simulink model "iopid_manually_tunning"  (R2017b)
settings: Solver=FixedStepAuto  StartTime=0.0  StopTime=100  FixedStep=0.01  RelTol=1e-3
undefined symbols (not defined in the file): CoordinateFrame, TypeMask, Velocity
libraries: robotlib x3, simulink x1
settings Model: Creator=bshang2  LastModifiedBy=bshang2
settings CodeAppCC: StateflowObjectComments=on

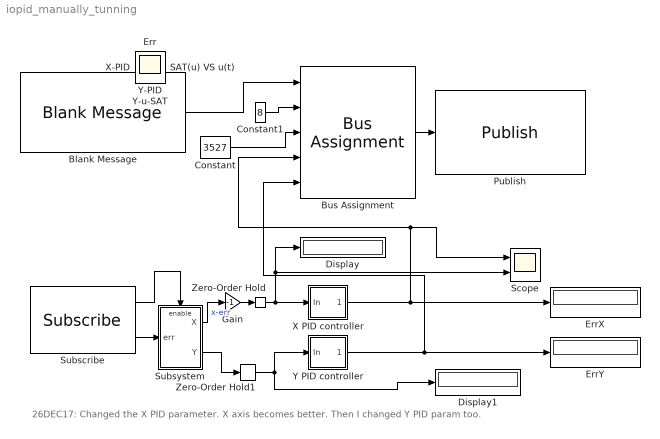
== system iopid_manually_tunning ==
  note: 26DEC17: Changed the X PID parameter. X axis becomes better. Then I changed Y PID param too.
  Blank Message : robotlib/Blank Message  SourceLibraryInfo=This block requires Robotics System Toolbox  messageType=mavros_msgs/PositionTarget  SampleTime=inf
      settings: SourceProductBaseCode=RO
  Bus Assignment : BusAssignment  AssignedSignals=CoordinateFrame,TypeMask,Velocity.X,Velocity.Y
  Constant : Constant  Value=3527  OutDataTypeStr=uint16
  Constant1 : Constant  Value=8  OutDataTypeStr=uint8
  Display : Display
  Display1 : Display
  ErrX : Display
  ErrY : Display
  Gain : Gain  Gain=-1
  Publish : robotlib/Publish  SourceLibraryInfo=This block requires Robotics System Toolbox  topicSource=Select from ROS network  topic=/mavros/setpoint_raw/local  messageType=mavros_msgs/PositionTarget  messageQueueLength=1
      settings: SourceProductBaseCode=RO
  Scope : Scope  NumInputPorts=2
  Subscribe : robotlib/Subscribe  SourceLibraryInfo=This block requires Robotics System Toolbox  topicSource=Select from ROS network  topic=/matlab/err  messageType=geometry_msgs/Pose2D  sampleTime=-1  messageQueueLength=1
      settings: SourceProductBaseCode=RO
  Subsystem : Subsystem
  X PID controller : Subsystem
  Y PID controller : Subsystem
  Zero-Order Hold : ZeroOrderHold  SampleTime=-1
  Zero-Order Hold1 : ZeroOrderHold  SampleTime=-1
  Err : Scope
  SAT(u) VS u(t) : Scope
  X-PID : Scope
  Y-PID : Scope
  Y-u-SAT : Scope
  wires:
  Blank Message/1 -> Bus Assignment/1
  X PID controller/1(Out) -> ErrX/1, Scope/1, Bus Assignment/4
  Bus Assignment/1 -> Publish/1
  Subscribe/2 -> Subsystem/1(err)
  Subsystem/1(X) -> Gain/1  "x-err"
  Subsystem/2(Y) -> Zero-Order Hold1/1
  Subscribe/1 -> Subsystem/Enable
  Y PID controller/1(Out) -> Bus Assignment/5, ErrY/1
  Constant/1 -> Bus Assignment/3
  Constant1/1 -> Bus Assignment/2
  Zero-Order Hold/1 -> Display/1, Scope/2, X PID controller/1(In)
  Zero-Order Hold1/1 -> Display1/1, Y PID controller/1(In)
  Gain/1 -> Zero-Order Hold/1

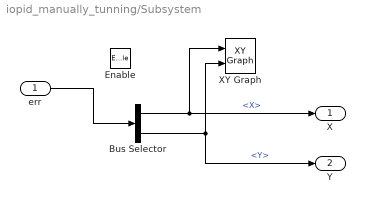
== system iopid_manually_tunning/Subsystem ==
  err : Inport
  Enable : EnablePort
  Bus Selector : BusSelector  OutputSignals=X,Y
  XY Graph : simulink/Sinks/XY Graph  xmin=-100  xmax=100  ymin=-100  ymax=100  st=-1
  X : Outport
  Y : Outport  Port=2
  wires:
  err/1 -> Bus Selector/1
  Bus Selector/1 -> X/1, XY Graph/1  "<X>"
  Bus Selector/2 -> Y/1, XY Graph/2  "<Y>"

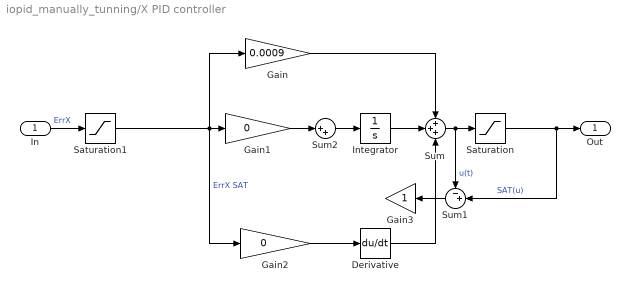
== system iopid_manually_tunning/X PID controller ==
  In : Inport
  Derivative : Derivative
  Gain : Gain  Gain=0.0009
  Gain1 : Gain  Gain=0
  Gain2 : Gain  Gain=0
  Gain3 : Gain
  Integrator : Integrator
  Saturation : Saturate  UpperLimit=0.3  LowerLimit=-0.3
  Saturation1 : Saturate  UpperLimit=100  LowerLimit=-100
  Sum : Sum  Inputs=+++
  Sum1 : Sum  Inputs=-+|
  Sum2 : Sum  Inputs=|++
  Out : Outport
  wires:
  Sum/1 -> Sum1/1, Saturation/1  "u(t)"
  In/1 -> Saturation1/1  "ErrX"
  Gain1/1 -> Sum2/1
  Gain2/1 -> Derivative/1
  Gain/1 -> Sum/1
  Integrator/1 -> Sum/2
  Derivative/1 -> Sum/3
  Saturation/1 -> Sum1/2, Out/1  "SAT(u)"
  Sum1/1 -> Gain3/1
  Sum2/1 -> Integrator/1
  Saturation1/1 -> Gain2/1, Gain1/1, Gain/1  "ErrX SAT"

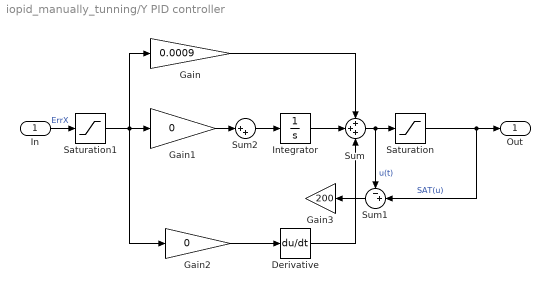
== system iopid_manually_tunning/Y PID controller ==
  In : Inport
  Derivative : Derivative
  Gain : Gain  Gain=0.0009
  Gain1 : Gain  Gain=0
  Gain2 : Gain  Gain=0
  Gain3 : Gain  Gain=200
  Integrator : Integrator
  Saturation : Saturate  UpperLimit=0.3  LowerLimit=-0.3
  Saturation1 : Saturate  UpperLimit=100  LowerLimit=-100
  Sum : Sum  Inputs=+++
  Sum1 : Sum  Inputs=-+|
  Sum2 : Sum  Inputs=|++
  Out : Outport
  wires:
  Sum/1 -> Sum1/1, Saturation/1  "u(t)"
  In/1 -> Saturation1/1  "ErrX"
  Gain1/1 -> Sum2/1
  Gain2/1 -> Derivative/1
  Gain/1 -> Sum/1
  Integrator/1 -> Sum/2
  Derivative/1 -> Sum/3
  Saturation/1 -> Sum1/2, Out/1  "SAT(u)"
  Sum1/1 -> Gain3/1
  Sum2/1 -> Integrator/1
  Saturation1/1 -> Gain/1, Gain1/1, Gain2/1
